simulink model "test_mashinka_mapp_4"  (R2020b)
settings: Solver=ode45  StartTime=0.0  StopTime=20000  RelTol=1e-3  EnableMultiTasking=on
undefined symbols (not defined in the file): CMD_ci_Re_9, CMD_fb, CMD_Firprg_0, CMD_Firprg_1, CMD_gain, CMD_ind_mult, CMD_ind_mult_1, CMD_ind_mult_2, CMD_ind_mult_3, CMD_ind_mult_4, CMD_ind_vol, CMD_ind_vol_1, CMD_ind_vol_2, CMD_ind_vol_3, CMD_ind_vol_4, CMD_nl, CMD_param_0, CMD_pedal, CMD_reset, CMD_shape_0, CMD_step_down, CMD_step_up, ind_mult_0, ind_mult_1, ind_mult_2, ind_mult_3, ind_mult_4, ind_mult_multiplier, num_harm_0, num_pts0, num_str0, num_str1, Res, rom_length
libraries: xbsIndex_r4 x2299
(part 2 of 11)

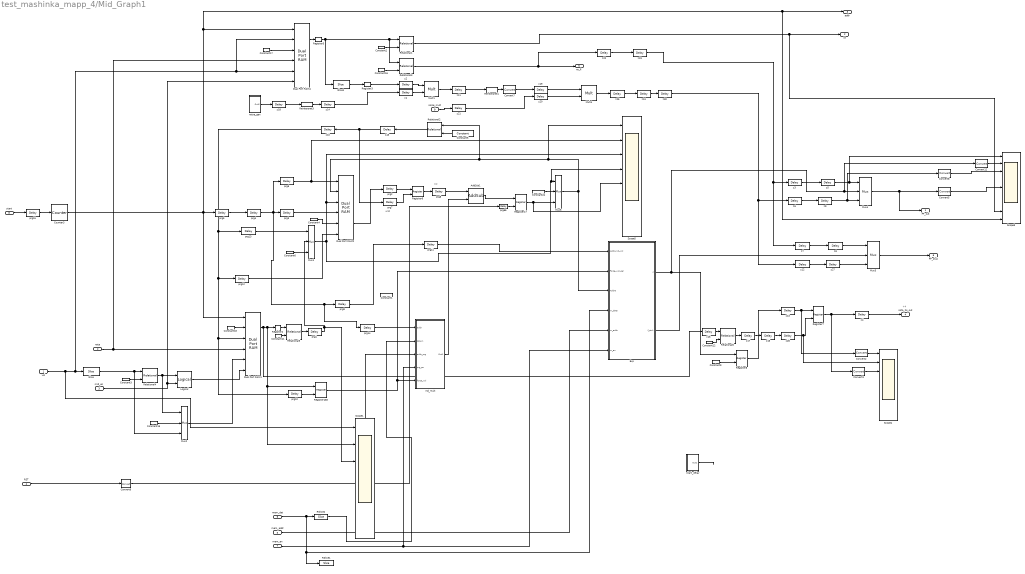
== system test_mashinka_mapp_4/Mid_Graph1 ==
  note: w90
  note: w2
  note: +4
  vol : Inport
  nota : Inport  Port=2
  mid_en : Inport  Port=3
  RST : Inport  Port=4
  mem_addr : Inport  Port=5
  mem_dat : Inport  Port=6
  mem_en : Inport  Port=7
  start : Inport  Port=8
  noise_mult : Inport  Port=9
  AddSub1 : xbsIndex_r4/AddSub  mode=Addition  use_carryin=off  use_carryout=off  en=off  latency=2  precision=User Defined  arith_type=Unsigned  n_bits=30  bin_pt=0  quantization=Truncate  overflow=Saturate  use_behavioral_HDL=off  hw_selection=Fabric  pipelined=off  dbl_ovrd=off  block_type=addsub
  Constant1 : xbsIndex_r4/Constant  const=4000  gui_display_data_type=Fixed-point  arith_type=Unsigned  n_bits=16  bin_pt=0  preci_type=Single  exp_width=8  frac_width=24  explicit_period=on  period=1  equ=P=C  opselect=C  inp2=PCIN>>17  opr=+  inp1=P  carry=CIN  dbl_ovrd=off  block_type=constant
      settings: block_version=VER_STRING_GOES_HERE
  Constant11 : xbsIndex_r4/Constant  const=1  gui_display_data_type=Fixed-point  arith_type=Unsigned  n_bits=7  bin_pt=0  preci_type=Single  exp_width=8  frac_width=24  explicit_period=on  period=1  equ=P=C  opselect=C  inp2=PCIN>>17  opr=+  inp1=P  carry=CIN  dbl_ovrd=off  block_type=constant
      settings: block_version=VER_STRING_GOES_HERE
  Constant{2,12,15,18} (4 alike) : xbsIndex_r4/Constant  const=0  gui_display_data_type=Fixed-point  arith_type=Unsigned  n_bits=7  bin_pt=0  preci_type=Single  exp_width=8  frac_width=24  explicit_period=on  period=1  equ=P=C  opselect=C  inp2=PCIN>>17  opr=+  inp1=P  carry=CIN  dbl_ovrd=off  block_type=constant
      settings: block_version=VER_STRING_GOES_HERE
  Constant16 : xbsIndex_r4/Constant  const=127  gui_display_data_type=Fixed-point  arith_type=Unsigned  n_bits=8  bin_pt=0  preci_type=Single  exp_width=8  frac_width=24  explicit_period=on  period=1  equ=P=C  opselect=C  inp2=PCIN>>17  opr=+  inp1=P  carry=CIN  dbl_ovrd=off  block_type=constant
      settings: block_version=VER_STRING_GOES_HERE
  Constant17 : xbsIndex_r4/Constant  const=0  gui_display_data_type=Fixed-point  arith_type=Boolean  n_bits=1  bin_pt=0  preci_type=Single  exp_width=8  frac_width=24  explicit_period=on  period=1  equ=P=C  opselect=C  inp2=PCIN>>17  opr=+  inp1=P  carry=CIN  dbl_ovrd=off  block_type=constant
      settings: block_version=VER_STRING_GOES_HERE
  Constant24 : xbsIndex_r4/Constant  const=0  gui_display_data_type=Fixed-point  arith_type=Unsigned  n_bits=30  bin_pt=0  preci_type=Single  exp_width=8  frac_width=24  explicit_period=on  period=1  equ=P=C  opselect=C  inp2=PCIN>>17  opr=+  inp1=P  carry=CIN  dbl_ovrd=off  block_type=constant
      settings: block_version=VER_STRING_GOES_HERE
  Constant3 : xbsIndex_r4/Constant  const=1  gui_display_data_type=Fixed-point  arith_type=Unsigned  n_bits=7  bin_pt=0  preci_type=Single  exp_width=8  frac_width=24  explicit_period=on  period=1  equ=P=C  opselect=C  inp2=PCIN>>17  opr=+  inp1=P  carry=CIN  dbl_ovrd=off  block_type=constant
      settings: block_version=VER_STRING_GOES_HERE
  Constant4 : xbsIndex_r4/Constant  const=0  gui_display_data_type=Fixed-point  arith_type=Unsigned  n_bits=30  bin_pt=0  preci_type=Single  exp_width=8  frac_width=24  explicit_period=on  period=1  equ=P=C  opselect=C  inp2=PCIN>>17  opr=+  inp1=P  carry=CIN  dbl_ovrd=off  block_type=constant
      settings: block_version=VER_STRING_GOES_HERE
  Constant5 : xbsIndex_r4/Constant  const=1000000000  gui_display_data_type=Fixed-point  arith_type=Unsigned  n_bits=30  bin_pt=0  preci_type=Single  exp_width=8  frac_width=24  explicit_period=off  period=1  equ=P=C  opselect=C  inp2=PCIN>>17  opr=+  inp1=P  carry=CIN  dbl_ovrd=off  block_type=constant
      settings: block_version=VER_STRING_GOES_HERE
  Constant6 : xbsIndex_r4/Constant  const=0  gui_display_data_type=Boolean  arith_type=Boolean  n_bits=24  bin_pt=0  preci_type=Single  exp_width=8  frac_width=24  explicit_period=on  period=1  equ=P=C  opselect=C  inp2=PCIN>>17  opr=+  inp1=P  carry=CIN  dbl_ovrd=off  block_type=constant
      settings: block_version=VER_STRING_GOES_HERE
  Constant9 : xbsIndex_r4/Constant  const=1  gui_display_data_type=Boolean  arith_type=Boolean  n_bits=24  bin_pt=0  preci_type=Single  exp_width=8  frac_width=24  explicit_period=on  period=1  equ=P=C  opselect=C  inp2=PCIN>>17  opr=+  inp1=P  carry=CIN  dbl_ovrd=off  block_type=constant
      settings: block_version=VER_STRING_GOES_HERE
  Convert{2..3,5,8,12} (5 alike) : xbsIndex_r4/Convert  gui_display_data_type=Floating-point  arith_type=Floating-point  n_bits=48  bin_pt=0  float_type=Single  exp_bits=8  fraction_bits=24  quantization="Round  (unbiased: +/- Inf)"  overflow=Saturate  en=off  latency=0  pipeline=off  dbl_ovrd=off  block_type=convert
  Convert6 : xbsIndex_r4/Convert  gui_display_data_type=Fixed-point  arith_type=Boolean  n_bits=48  bin_pt=48  float_type=Single  exp_bits=8  fraction_bits=24  quantization=Truncate  overflow=Saturate  en=off  latency=0  pipeline=off  dbl_ovrd=off  block_type=convert
      settings: xl_area=[0 0 0 0 0 0 0]  block_version=8.2-EVAL
  Convert7 : xbsIndex_r4/Convert  gui_display_data_type=Floating-point  arith_type=Floating-point  n_bits=48  bin_pt=0  float_type=Single  exp_bits=8  fraction_bits=24  quantization="Round  (unbiased: +/- Inf)"  overflow=Saturate  en=off  latency=6  pipeline=off  dbl_ovrd=off  block_type=convert
  Counter3 : xbsIndex_r4/Counter  cnt_type=Count Limited  cnt_to=95  operation=Up  start_count=0  cnt_by_val=1  arith_type=Unsigned  n_bits=7  bin_pt=0  load_pin=off  rst=off  en=on  explicit_period=on  period=1  use_behavioral_HDL=off  implementation=Fabric  use_rpm=off  dbl_ovrd=off  block_type=counter
      settings: block_version=8.2.02
  Dual Port RAM1 : xbsIndex_r4/Dual Port RAM  depth=96  initVector=zeros  distributed_mem=Block RAM  init_a=0  init_b=0  rst_a=off  rst_b=off  en_a=off  en_b=off  latency=1  write_mode_A=Read Before Write  write_mode_B=Read After Write  optimize=Area  dbl_ovrd=off  simulation_type=fast_sim  block_type=dpram
      settings: block_version=10.1.1
  Dual Port RAM2 : xbsIndex_r4/Dual Port RAM  depth=96  initVector=zeros  distributed_mem=Block RAM  init_a=0  init_b=0  rst_a=off  rst_b=off  en_a=off  en_b=off  latency=1  write_mode_A=Read Before Write  write_mode_B=Read After Write  optimize=Area  dbl_ovrd=off  simulation_type=fast_sim  block_type=dpram
      settings: block_version=10.1.1
  Dual Port RAM4 : xbsIndex_r4/Dual Port RAM  depth=96  initVector=zeros  distributed_mem=Block RAM  init_a=0  init_b=0  rst_a=off  rst_b=off  en_a=off  en_b=off  latency=1  write_mode_A=Read Before Write  write_mode_B=Read After Write  optimize=Area  dbl_ovrd=off  simulation_type=fast_sim  block_type=dpram
      settings: block_version=10.1.1
  Exp : Subsystem
  Logical : xbsIndex_r4/Logical  logical_function=AND  inputs=2  en=off  latency=0  precision=Full  arith_type=Unsigned  n_bits=16  bin_pt=0  align_bp=on  dbl_ovrd=off  block_type=logical
  Mult1 : xbsIndex_r4/Mult  precision=Full  arith_type="Signed  (2's comp)"  n_bits=16  bin_pt=14  quantization=Truncate  overflow=Wrap  en=off  latency=6  use_behavioral_HDL=off  opt=Speed  use_embedded=on  optimum_pipeline=off  pipeline=on  dbl_ovrd=off  use_rpm=on  placement_style=Triangular  block_type=mult
  Mult4 : xbsIndex_r4/Mult  precision=Full  arith_type="Signed  (2's comp)"  n_bits=16  bin_pt=14  quantization=Truncate  overflow=Wrap  en=off  latency=6  use_behavioral_HDL=off  opt=Speed  use_embedded=on  optimum_pipeline=off  pipeline=on  dbl_ovrd=off  use_rpm=on  placement_style=Triangular  block_type=mult
  Mux{1..5} (5 alike) : xbsIndex_r4/Mux  inputs=2  en=off  latency=0  precision=Full  arith_type=Unsigned  n_bits=16  bin_pt=14  quantization=Truncate  overflow=Wrap  dbl_ovrd=off  block_type=mux
  RSlice1 : xbsIndex_r4/Slice  nbits=30  boolean_output=off  mode=Lower Bit Location + Width  bit1=0  base1=MSB of Input  bit0=0  base0=LSB of Input  dbl_ovrd=off  block_type=slice
      settings: block_version=VER_STRING_GOES_HERE
  RSlice2 : xbsIndex_r4/Slice  nbits=24  boolean_output=off  mode=Lower Bit Location + Width  bit1=0  base1=MSB of Input  bit0=0  base0=LSB of Input  dbl_ovrd=off  block_type=slice
      settings: block_version=VER_STRING_GOES_HERE
  Register17 : xbsIndex_r4/Register  init=0  rst=on  en=off  dbl_ovrd=off  block_type=register
  Register183 : xbsIndex_r4/Register  init=0  rst=on  en=off  dbl_ovrd=off  block_type=register
  Register2 : xbsIndex_r4/Register  init=0  rst=off  en=off  dbl_ovrd=off  block_type=register
  Register3 : xbsIndex_r4/Register  init=0  rst=off  en=off  dbl_ovrd=off  block_type=register
  Register5 : xbsIndex_r4/Register  init=0  rst=off  en=off  dbl_ovrd=off  block_type=register
  Register6 : xbsIndex_r4/Register  init=0  rst=on  en=off  dbl_ovrd=off  block_type=register
  Register7 : xbsIndex_r4/Register  init=1  rst=off  en=on  dbl_ovrd=off  block_type=register
  Register8 : xbsIndex_r4/Register  init=0  rst=off  en=on  dbl_ovrd=off  block_type=register
  Reinterpret1 : xbsIndex_r4/Reinterpret  force_arith_type=on  arith_type="Signed  (2's comp)"  force_bin_pt=on  bin_pt=30  block_type=reinterpret
  Reinterpret3 : xbsIndex_r4/Reinterpret  force_arith_type=on  arith_type="Signed  (2's comp)"  force_bin_pt=on  bin_pt=0  block_type=reinterpret
  Relational{1,3..6} (5 alike) : xbsIndex_r4/Relational  mode=a>b  op_type=Bool  en=off  latency=0  dbl_ovrd=off  block_type=relational
  Relational2 : xbsIndex_r4/Relational  mode=a>=b  op_type=Bool  en=off  latency=0  dbl_ovrd=off  block_type=relational
  Scope1 : Scope  NumInputPorts=7
  Scope3 : Scope  NumInputPorts=9
  Scope4 : Scope  NumInputPorts=8
  Scope5 : Scope  NumInputPorts=8
  Slice : xbsIndex_r4/Slice  nbits=7  boolean_output=off  mode=Lower Bit Location + Width  bit1=0  base1=MSB of Input  bit0=0  base0=LSB of Input  dbl_ovrd=off  block_type=slice
  Slice1 : xbsIndex_r4/Slice  nbits=7  boolean_output=off  mode=Lower Bit Location + Width  bit1=0  base1=MSB of Input  bit0=0  base0=LSB of Input  dbl_ovrd=off  block_type=slice
  ind_mult : Subsystem
  noise_gen : Subsystem
  prg1 : xbsIndex_r4/Delay  rst=off  infoeditControl=Selection of Reset will increase slice count due to use of real FFs and instead of SRLs  en=off  latency=12  reg_retiming=on  dbl_ovrd=off  block_type=delay
      settings: block_version=8.2-EVAL
  prg10 : xbsIndex_r4/Delay  rst=off  infoeditControl=Selection of Reset will increase slice count due to use of real FFs and instead of SRLs  en=off  latency=8  reg_retiming=on  dbl_ovrd=off  block_type=delay
      settings: block_version=8.2-EVAL
  prg11 : xbsIndex_r4/Delay  rst=off  infoeditControl=Selection of Reset will increase slice count due to use of real FFs and instead of SRLs  en=off  latency=2  reg_retiming=on  dbl_ovrd=off  block_type=delay
      settings: block_version=8.2-EVAL
  prg12 : xbsIndex_r4/Delay  rst=off  infoeditControl=Selection of Reset will increase slice count due to use of real FFs and instead of SRLs  en=off  latency=6  reg_retiming=on  dbl_ovrd=off  block_type=delay
      settings: block_version=8.2-EVAL
  prg13 : xbsIndex_r4/Delay  rst=off  infoeditControl=Selection of Reset will increase slice count due to use of real FFs and instead of SRLs  en=off  latency=14  reg_retiming=on  dbl_ovrd=off  block_type=delay
      settings: block_version=8.2-EVAL
  prg14 : xbsIndex_r4/Delay  rst=off  infoeditControl=Selection of Reset will increase slice count due to use of real FFs and instead of SRLs  en=off  latency=6  reg_retiming=on  dbl_ovrd=off  block_type=delay
      settings: block_version=8.2-EVAL
  prg{2,4,15,66} (4 alike) : xbsIndex_r4/Delay  rst=off  infoeditControl=Selection of Reset will increase slice count due to use of real FFs and instead of SRLs  en=off  latency=1  reg_retiming=on  dbl_ovrd=off  block_type=delay
      settings: block_version=8.2-EVAL
  prg3 : xbsIndex_r4/Delay  rst=off  infoeditControl=Selection of Reset will increase slice count due to use of real FFs and instead of SRLs  en=off  latency=8 + 7  reg_retiming=on  dbl_ovrd=off  block_type=delay
      settings: block_version=8.2-EVAL
  prg5 : xbsIndex_r4/Delay  rst=off  infoeditControl=Selection of Reset will increase slice count due to use of real FFs and instead of SRLs  en=off  latency=86  reg_retiming=on  dbl_ovrd=off  block_type=delay
      settings: block_version=8.2-EVAL
  prg6 : xbsIndex_r4/Delay  rst=off  infoeditControl=Selection of Reset will increase slice count due to use of real FFs and instead of SRLs  en=off  latency=16 + 7  reg_retiming=on  dbl_ovrd=off  block_type=delay
      settings: block_version=8.2-EVAL
  prg7 : xbsIndex_r4/Delay  rst=off  infoeditControl=Selection of Reset will increase slice count due to use of real FFs and instead of SRLs  en=off  latency=93 - 6  reg_retiming=on  dbl_ovrd=off  block_type=delay
      settings: block_version=8.2-EVAL
  prg8 : xbsIndex_r4/Delay  rst=off  infoeditControl=Selection of Reset will increase slice count due to use of real FFs and instead of SRLs  en=off  latency=2  reg_retiming=on  dbl_ovrd=off  block_type=delay
      settings: block_version=8.2-EVAL
  prg9 : xbsIndex_r4/Delay  rst=off  infoeditControl=Selection of Reset will increase slice count due to use of real FFs and instead of SRLs  en=off  latency=8  reg_retiming=on  dbl_ovrd=off  block_type=delay
      settings: block_version=8.2-EVAL
  start_delay : Subsystem
  z{1..2,4..5,8..9,11,13..14,16..21,23,25..27,30} (20 alike) : xbsIndex_r4/Delay  rst=off  infoeditControl=Selection of Reset will increase slice count due to use of real FFs and instead of SRLs  en=off  latency=1  reg_retiming=on  dbl_ovrd=off  block_type=delay
      settings: block_version=8.2-EVAL
  z10 : xbsIndex_r4/Delay  rst=off  infoeditControl=Selection of Reset will increase slice count due to use of real FFs and instead of SRLs  en=off  latency=86 -7  reg_retiming=on  dbl_ovrd=off  block_type=delay
      settings: block_version=8.2-EVAL
  z{3,6..7,12} (4 alike) : xbsIndex_r4/Delay  rst=off  infoeditControl=Selection of Reset will increase slice count due to use of real FFs and instead of SRLs  en=off  latency=35 + 7  reg_retiming=on  dbl_ovrd=off  block_type=delay
      settings: block_version=8.2-EVAL
  z15 : xbsIndex_r4/Delay  rst=off  infoeditControl=Selection of Reset will increase slice count due to use of real FFs and instead of SRLs  en=off  latency=98  reg_retiming=on  dbl_ovrd=off  block_type=delay
      settings: block_version=8.2-EVAL
  z22 : xbsIndex_r4/Delay  rst=off  infoeditControl=Selection of Reset will increase slice count due to use of real FFs and instead of SRLs  en=off  latency=54  reg_retiming=on  dbl_ovrd=off  block_type=delay
      settings: block_version=8.2-EVAL
  z24 : xbsIndex_r4/Delay  rst=off  infoeditControl=Selection of Reset will increase slice count due to use of real FFs and instead of SRLs  en=off  latency=31  reg_retiming=on  dbl_ovrd=off  block_type=delay
      settings: block_version=8.2-EVAL
  z43 : xbsIndex_r4/Delay  rst=off  infoeditControl=Selection of Reset will increase slice count due to use of real FFs and instead of SRLs  en=off  latency=3  reg_retiming=on  dbl_ovrd=off  block_type=delay
      settings: block_version=8.2-EVAL
  FF_out : Outport  VectorParamsAs1DForOutWhenUnconnected=off
  nn : Outport  Port=2  VectorParamsAs1DForOutWhenUnconnected=off
  addr : Outport  Port=3  VectorParamsAs1DForOutWhenUnconnected=off
  nota_24_out : Outport  Port=4  VectorParamsAs1DForOutWhenUnconnected=off
  nn_fl : Outport  Port=5  VectorParamsAs1DForOutWhenUnconnected=off
  FF_stuk : Outport  Port=6  VectorParamsAs1DForOutWhenUnconnected=off
  wires:
  z5/1 -> Mux4/1, Scope3/1
  Convert3/1 -> Scope4/3
  Convert2/1 -> Scope4/1
  Constant12/1 -> Relational6/2
  Constant9/1 -> Register8/2
  z13/1 -> Register7/1, Convert2/1
  Relational6/1 -> z17/1
  z15/1 -> z26/1
  z16/1 -> Relational6/1
  z17/1 -> z15/1
  z26/1 -> Register7/2, Scope4/2
  Register8/1 -> z13/1
  Convert12/1 -> Scope3/2
  Convert8/1 -> Scope3/3
  Convert5/1 -> Scope3/5
  Mux4/1 -> Convert5/1, FF_out/1
  z9/1 -> Mux4/3, Convert8/1
  z3/1 -> z5/1
  Counter3/1 -> prg5/1, Dual Port RAM1/1, addr/1, Scope3/9, Dual Port RAM4/1
  mem_dat/1 -> RSlice2/1, RSlice1/1, Exp/4(m_data)
  Exp/1(f) -> Mux4/2, Convert12/1, Register8/1
  z30/1 -> z12/1, z6/1
  z25/1 -> z24/1
  z24/1 -> z30/1
  z23/1 -> z7/1, z3/1
  z22/1 -> z23/1
  Mult4/1 -> z25/1
  z21/1 -> z20/1
  noise_mult/1 -> z21/1
  Mult1/1 -> z11/1
  z19/1 -> Mult4/1
  z11/1 -> Reinterpret1/1
  Convert7/1 -> z19/1
  Reinterpret1/1 -> Convert7/1
  z20/1 -> Mult4/2
  Register3/1 -> z2/1
  z2/1 -> Mult1/1
  z1/1 -> Mult1/2
  Slice1/1 -> Register3/1
  Reinterpret3/1 -> z14/1
  z14/1 -> z1/1
  Relational3/1 -> nn_fl/1, z22/1
  Constant16/1 -> Relational3/2
  vol/1 -> Slice/1, Dual Port RAM4/5, Dual Port RAM4/2, Scope1/1
  Slice/1 -> Mux2/3, Relational4/1
  prg3/1 -> Dual Port RAM2/4
  prg1/1 -> Mux1/2, Scope1/3
  Constant6/1 -> Mux1/3
  prg13/1 -> Mux1/1
  Constant4/1 -> Dual Port RAM2/5
  prg12/1 -> Dual Port RAM2/6
  z4/1 -> nota_24_out/1
  prg5/1 -> prg4/1
  Logical/1 -> Dual Port RAM1/6
  prg11/1 -> Exp/1(Addr_ind_vol)
  z10/1 -> prg12/1, Dual Port RAM1/3, prg10/1, prg13/1
  Dual Port RAM1/1 -> Register2/1, Register183/1, Scope1/2, z16/1
  Relational5/1 -> prg1/1
  prg4/1 -> prg14/1, prg9/1, prg3/1, prg6/1
  prg6/1 -> Dual Port RAM2/1, Scope5/2
  Register5/1 -> Relational1/1, Relational3/1, Slice1/1
  prg2/1 -> Register6/1
  Dual Port RAM2/2 -> prg2/1
  Constant17/1 -> Dual Port RAM4/3
  Dual Port RAM4/1 -> Register5/1
  Register6/1 -> prg8/1
  Constant18/1 -> Dual Port RAM1/2
  prg7/1 -> Register6/2
  prg10/1 -> Register183/2
  Constant2/1 -> Relational1/2
  Relational1/1 -> nn/1, Scope3/8
  Constant5/1 -> Relational2/2
  z43/1 -> z10/1, prg7/1
  Relational2/1 -> z43/1
  Constant3/1 -> Relational4/2
  Relational4/1 -> Mux2/1, Logical/1
  Constant11/1 -> Relational5/2
  Register2/1 -> Relational5/1
  AddSub1/1 -> Register17/1
  RST/1 -> Convert6/1
  Convert6/1 -> prg66/1
  prg66/1 -> Register17/2
  Mux5/1 -> Scope5/1, Relational2/1, Dual Port RAM2/2, Exp/3(Addr0)
  Register17/1 -> Mux5/3, Scope5/5
  Constant24/1 -> Mux5/2
  Mux1/1 -> Dual Port RAM2/3, Scope5/3, Mux5/1, Scope5/4
  mem_en/1 -> Exp/6(m_en), ind_mult/4(prg_en)
  mem_addr/1 -> Exp/5(m_addr), ind_mult/3(addr_prg)
  RSlice2/1 -> ind_mult/2(dat_in)
  Register183/1 -> Exp/2(Force_vol_sel), ind_mult/5(force_vol)
  ind_mult/1(Out1) -> AddSub1/2
  prg9/1 -> prg11/1
  prg8/1 -> AddSub1/1
  start_delay/1(Out1) -> ?
  prg14/1 -> ind_mult/1(addr)
  start/1 -> prg15/1
  prg15/1 -> Counter3/1
  mid_en/1 -> Dual Port RAM4/6, Logical/2
  nota/1 -> Dual Port RAM4/4, Dual Port RAM1/4
  z18/1 -> Reinterpret3/1
  Constant15/1 -> Mux2/2
  Mux2/1 -> Dual Port RAM1/5
  noise_gen/1(Out2) -> z18/1
  Register7/1 -> z4/1, Convert3/1
  z6/1 -> z9/1
  z12/1 -> z27/1
  Exp/2(f_stuk) -> Mux3/2
  z7/1 -> z8/1
  z27/1 -> Mux3/3
  Mux3/1 -> FF_stuk/1
  z8/1 -> Mux3/1

== system test_mashinka_mapp_4/Reciever16 ==
  s_dat : Inport
  clk : Inport  Port=2
  frm : Inport  Port=3
  Convert : xbsIndex_r4/Convert  gui_display_data_type=Fixed-point  arith_type=Boolean  n_bits=16  bin_pt=14  float_type=Single  exp_bits=8  fraction_bits=24  quantization=Truncate  overflow=Wrap  en=off  latency=0  pipeline=off  dbl_ovrd=off  block_type=convert
      settings: xl_area=[0 0 0 0 0 0 0]  block_version=8.2-EVAL
  Convert1 : xbsIndex_r4/Convert  gui_display_data_type=Boolean  arith_type=Boolean  n_bits=16  bin_pt=14  float_type=Single  exp_bits=8  fraction_bits=24  quantization=Truncate  overflow=Wrap  en=off  latency=0  pipeline=off  dbl_ovrd=off  block_type=convert
      settings: xl_area=[0 0 0 0 0 0 0]  block_version=8.2-EVAL
  Delay : xbsIndex_r4/Delay  rst=off  infoeditControl=Selection of Reset will increase slice count due to use of real FFs and instead of SRLs  en=off  latency=1  reg_retiming=on  dbl_ovrd=off  block_type=delay
      settings: infoedit=Hardware notes: A delay line is a chain, each link of which is an SRL16 followed by a flip-flop. If register retiming is enabled, the delay line is a chain of flip-flops.  xl_area=[1 1 0 0 0 0 0]  block_version=8.2-EVAL
  Delay1 : xbsIndex_r4/Delay  rst=off  infoeditControl=Selection of Reset will increase slice count due to use of real FFs and instead of SRLs  en=off  latency=5  reg_retiming=on  dbl_ovrd=off  block_type=delay
      settings: infoedit=Hardware notes: A delay line is a chain, each link of which is an SRL16 followed by a flip-flop. If register retiming is enabled, the delay line is a chain of flip-flops.  xl_area=[1 1 0 1 0 0 0]  block_version=8.2-EVAL
  Delay2 : xbsIndex_r4/Delay  rst=off  infoeditControl=Selection of Reset will increase slice count due to use of real FFs and instead of SRLs  en=off  latency=1  reg_retiming=on  dbl_ovrd=off  block_type=delay
      settings: infoedit=Hardware notes: A delay line is a chain, each link of which is an SRL16 followed by a flip-flop. If register retiming is enabled, the delay line is a chain of flip-flops.  xl_area=[1 1 0 0 0 0 0]  block_version=8.2-EVAL
  Delay3 : xbsIndex_r4/Delay  rst=off  infoeditControl=Selection of Reset will increase slice count due to use of real FFs and instead of SRLs  en=off  latency=7  reg_retiming=on  dbl_ovrd=off  block_type=delay
      settings: infoedit=Hardware notes: A delay line is a chain, each link of which is an SRL16 followed by a flip-flop. If register retiming is enabled, the delay line is a chain of flip-flops.  xl_area=[1 1 0 1 0 0 0]  block_version=8.2-EVAL
  Delay4 : xbsIndex_r4/Delay  rst=off  infoeditControl=Selection of Reset will increase slice count due to use of real FFs and instead of SRLs  en=off  latency=3  reg_retiming=on  dbl_ovrd=off  block_type=delay
      settings: infoedit=Hardware notes: A delay line is a chain, each link of which is an SRL16 followed by a flip-flop. If register retiming is enabled, the delay line is a chain of flip-flops.  xl_area=[1 1 0 0 0 0 0]  block_version=8.2-EVAL
  Delay5 : xbsIndex_r4/Delay  rst=off  infoeditControl=Selection of Reset will increase slice count due to use of real FFs and instead of SRLs  en=off  latency=1  reg_retiming=on  dbl_ovrd=off  block_type=delay
      settings: infoedit=Hardware notes: A delay line is a chain, each link of which is an SRL16 followed by a flip-flop. If register retiming is enabled, the delay line is a chain of flip-flops.  xl_area=[1 1 0 0 0 0 0]  block_version=8.2-EVAL
  Inverter : xbsIndex_r4/Inverter  en=off  latency=0  dbl_ovrd=off  block_type=inv
      settings: xl_area=[0 0 0 0 0 0 0]  block_version=8.2-EVAL
  Logical : xbsIndex_r4/Logical  logical_function=XOR  inputs=2  en=off  latency=0  precision=Full  arith_type=Unsigned  n_bits=16  bin_pt=0  align_bp=on  dbl_ovrd=off  block_type=logical
      settings: xl_area=[1 0 0 1 0 0 0]  block_version=8.2-EVAL
  Logical1 : xbsIndex_r4/Logical  logical_function=AND  inputs=2  en=off  latency=0  precision=Full  arith_type=Unsigned  n_bits=16  bin_pt=0  align_bp=on  dbl_ovrd=off  block_type=logical
      settings: xl_area=[1 0 0 1 0 0 0]  block_version=8.2-EVAL
  Scope : Scope  NumInputPorts=4
  Subsystem1 : Subsystem
  Z1 : Subsystem
  Out1 : Outport  VectorParamsAs1DForOutWhenUnconnected=off
  reset_z1 : Outport  Port=2  VectorParamsAs1DForOutWhenUnconnected=off
  wires:
  frm/1 -> Delay3/1
  clk/1 -> Delay2/1
  s_dat/1 -> Delay1/1
  Delay/1 -> Logical/1
  Logical/1 -> Logical1/1
  Logical1/1 -> Convert/1
  Convert/1 -> Scope/3, Subsystem1/2(en), Delay4/1, Delay5/1
  Delay1/1 -> Scope/1, Subsystem1/1(data)
  Delay2/1 -> Z1/1(In1)
  Convert1/1 -> Scope/2, Subsystem1/3(clock)
  Z1/1(Out1) -> Convert1/1
  Inverter/1 -> Logical1/2
  Delay3/1 -> Logical/2, Inverter/1, Delay/1
  Delay4/1 -> Subsystem1/4(reset)
  Subsystem1/1(Out1) -> Scope/4, Out1/1
  Delay5/1 -> reset_z1/1

== system test_mashinka_mapp_4/Reciever50 ==
  s_dat : Inport
  clk : Inport  Port=2
  frm : Inport  Port=3
  Convert : xbsIndex_r4/Convert  gui_display_data_type=Fixed-point  arith_type=Boolean  n_bits=16  bin_pt=14  float_type=Single  exp_bits=8  fraction_bits=24  quantization=Truncate  overflow=Wrap  en=off  latency=0  pipeline=off  dbl_ovrd=off  block_type=convert
      settings: xl_area=[0 0 0 0 0 0 0]  block_version=8.2-EVAL
  Convert1 : xbsIndex_r4/Convert  gui_display_data_type=Boolean  arith_type=Boolean  n_bits=16  bin_pt=14  float_type=Single  exp_bits=8  fraction_bits=24  quantization=Truncate  overflow=Wrap  en=off  latency=0  pipeline=off  dbl_ovrd=off  block_type=convert
      settings: xl_area=[0 0 0 0 0 0 0]  block_version=8.2-EVAL
  Delay : xbsIndex_r4/Delay  rst=off  infoeditControl=Selection of Reset will increase slice count due to use of real FFs and instead of SRLs  en=off  latency=1  reg_retiming=on  dbl_ovrd=off  block_type=delay
      settings: infoedit=Hardware notes: A delay line is a chain, each link of which is an SRL16 followed by a flip-flop. If register retiming is enabled, the delay line is a chain of flip-flops.  xl_area=[1 1 0 0 0 0 0]  block_version=8.2-EVAL
  Delay1 : xbsIndex_r4/Delay  rst=off  infoeditControl=Selection of Reset will increase slice count due to use of real FFs and instead of SRLs  en=off  latency=5  reg_retiming=on  dbl_ovrd=off  block_type=delay
      settings: infoedit=Hardware notes: A delay line is a chain, each link of which is an SRL16 followed by a flip-flop. If register retiming is enabled, the delay line is a chain of flip-flops.  xl_area=[1 1 0 1 0 0 0]  block_version=8.2-EVAL
  Delay2 : xbsIndex_r4/Delay  rst=off  infoeditControl=Selection of Reset will increase slice count due to use of real FFs and instead of SRLs  en=off  latency=1  reg_retiming=on  dbl_ovrd=off  block_type=delay
      settings: infoedit=Hardware notes: A delay line is a chain, each link of which is an SRL16 followed by a flip-flop. If register retiming is enabled, the delay line is a chain of flip-flops.  xl_area=[1 1 0 0 0 0 0]  block_version=8.2-EVAL
  Delay3 : xbsIndex_r4/Delay  rst=off  infoeditControl=Selection of Reset will increase slice count due to use of real FFs and instead of SRLs  en=off  latency=7  reg_retiming=on  dbl_ovrd=off  block_type=delay
      settings: infoedit=Hardware notes: A delay line is a chain, each link of which is an SRL16 followed by a flip-flop. If register retiming is enabled, the delay line is a chain of flip-flops.  xl_area=[1 1 0 1 0 0 0]  block_version=8.2-EVAL
  Delay4 : xbsIndex_r4/Delay  rst=off  infoeditControl=Selection of Reset will increase slice count due to use of real FFs and instead of SRLs  en=off  latency=3  reg_retiming=on  dbl_ovrd=off  block_type=delay
      settings: infoedit=Hardware notes: A delay line is a chain, each link of which is an SRL16 followed by a flip-flop. If register retiming is enabled, the delay line is a chain of flip-flops.  xl_area=[1 1 0 0 0 0 0]  block_version=8.2-EVAL
  Delay5 : xbsIndex_r4/Delay  rst=off  infoeditControl=Selection of Reset will increase slice count due to use of real FFs and instead of SRLs  en=off  latency=1  reg_retiming=on  dbl_ovrd=off  block_type=delay
      settings: infoedit=Hardware notes: A delay line is a chain, each link of which is an SRL16 followed by a flip-flop. If register retiming is enabled, the delay line is a chain of flip-flops.  xl_area=[1 1 0 0 0 0 0]  block_version=8.2-EVAL
  Inverter : xbsIndex_r4/Inverter  en=off  latency=0  dbl_ovrd=off  block_type=inv
      settings: xl_area=[0 0 0 0 0 0 0]  block_version=8.2-EVAL
  Logical : xbsIndex_r4/Logical  logical_function=XOR  inputs=2  en=off  latency=0  precision=Full  arith_type=Unsigned  n_bits=16  bin_pt=0  align_bp=on  dbl_ovrd=off  block_type=logical
      settings: xl_area=[1 0 0 1 0 0 0]  block_version=8.2-EVAL
  Logical1 : xbsIndex_r4/Logical  logical_function=AND  inputs=2  en=off  latency=0  precision=Full  arith_type=Unsigned  n_bits=16  bin_pt=0  align_bp=on  dbl_ovrd=off  block_type=logical
      settings: xl_area=[1 0 0 1 0 0 0]  block_version=8.2-EVAL
  Scope : Scope  NumInputPorts=4
  Subsystem1 : Subsystem
  Z1 : Subsystem
  Out1 : Outport  VectorParamsAs1DForOutWhenUnconnected=off
  reset_z1 : Outport  Port=2  VectorParamsAs1DForOutWhenUnconnected=off
  wires:
  Delay5/1 -> reset_z1/1
  Subsystem1/1(Out1) -> Out1/1, Scope/4
  Delay4/1 -> Subsystem1/4(reset)
  Delay3/1 -> Delay/1, Inverter/1, Logical/2
  Inverter/1 -> Logical1/2
  Z1/1(Out1) -> Convert1/1
  Convert1/1 -> Subsystem1/3(clock), Scope/2
  Delay2/1 -> Z1/1(In1)
  Delay1/1 -> Subsystem1/1(data), Scope/1
  Convert/1 -> Delay5/1, Delay4/1, Subsystem1/2(en), Scope/3
  Logical1/1 -> Convert/1
  Logical/1 -> Logical1/1
  Delay/1 -> Logical/1
  s_dat/1 -> Delay1/1
  clk/1 -> Delay2/1
  frm/1 -> Delay3/1

== system test_mashinka_mapp_4/SIMULATION ==
  Accumulator : xbsIndex_r4/Accumulator  operation=Add  n_bits=3  overflow=Wrap  scale=1  rst=off  hasbypass=off  infoeditControl=reset for floating point data type must be asserted for a minimum of 2 cycles  en=on  latency=1  msb_inp=100  msb=100  lsb=-100  use_behavioral_HDL=on  implementation=Fabric  dbl_ovrd=off  block_type=accum
      settings: block_version=11.4
  Concat{1..6} (6 alike) : xbsIndex_r4/Concat  num_inputs=2  dbl_ovrd=off  block_type=concat
  Constant1 : xbsIndex_r4/Constant  const=60000  gui_display_data_type=Fixed-point  arith_type=Unsigned  n_bits=18  bin_pt=0  preci_type=Single  exp_width=8  frac_width=24  explicit_period=on  period=1  equ=P=C  opselect=C  inp2=PCIN>>17  opr=+  inp1=P  carry=CIN  dbl_ovrd=off  block_type=constant
      settings: block_version=8.2-EVAL
  Constant10 : xbsIndex_r4/Constant  const=1  gui_display_data_type=Boolean  arith_type=Boolean  n_bits=18  bin_pt=0  preci_type=Single  exp_width=8  frac_width=24  explicit_period=on  period=1  equ=P=C  opselect=C  inp2=PCIN>>17  opr=+  inp1=P  carry=CIN  dbl_ovrd=off  block_type=constant
      settings: block_version=8.2-EVAL
  Constant2 : xbsIndex_r4/Constant  const=700000  gui_display_data_type=Fixed-point  arith_type=Unsigned  n_bits=18  bin_pt=0  preci_type=Single  exp_width=8  frac_width=24  explicit_period=on  period=1  equ=P=C  opselect=C  inp2=PCIN>>17  opr=+  inp1=P  carry=CIN  dbl_ovrd=off  block_type=constant
      settings: block_version=8.2-EVAL
  Constant3 : xbsIndex_r4/Constant  const=1500  gui_display_data_type=Fixed-point  arith_type=Unsigned  n_bits=18  bin_pt=0  preci_type=Single  exp_width=8  frac_width=24  explicit_period=on  period=1  equ=P=C  opselect=C  inp2=PCIN>>17  opr=+  inp1=P  carry=CIN  dbl_ovrd=off  block_type=constant
      settings: block_version=8.2-EVAL
  Constant4 : xbsIndex_r4/Constant  const=1  gui_display_data_type=Fixed-point  arith_type=Unsigned  n_bits=1  bin_pt=0  preci_type=Single  exp_width=8  frac_width=24  explicit_period=on  period=1  equ=P=C  opselect=C  inp2=PCIN>>17  opr=+  inp1=P  carry=CIN  dbl_ovrd=off  block_type=constant
      settings: block_version=8.2-EVAL
  Constant5 : xbsIndex_r4/Constant  const=1500  gui_display_data_type=Fixed-point  arith_type=Unsigned  n_bits=18  bin_pt=0  preci_type=Single  exp_width=8  frac_width=24  explicit_period=on  period=1  equ=P=C  opselect=C  inp2=PCIN>>17  opr=+  inp1=P  carry=CIN  dbl_ovrd=off  block_type=constant
      settings: block_version=8.2-EVAL
  Constant6 : xbsIndex_r4/Constant  const=2000  gui_display_data_type=Fixed-point  arith_type=Unsigned  n_bits=18  bin_pt=0  preci_type=Single  exp_width=8  frac_width=24  explicit_period=on  period=1  equ=P=C  opselect=C  inp2=PCIN>>17  opr=+  inp1=P  carry=CIN  dbl_ovrd=off  block_type=constant
      settings: block_version=8.2-EVAL
  Constant7 : xbsIndex_r4/Constant  const=2500  gui_display_data_type=Fixed-point  arith_type=Unsigned  n_bits=18  bin_pt=0  preci_type=Single  exp_width=8  frac_width=24  explicit_period=on  period=1  equ=P=C  opselect=C  inp2=PCIN>>17  opr=+  inp1=P  carry=CIN  dbl_ovrd=off  block_type=constant
      settings: block_version=8.2-EVAL
  Constant8 : xbsIndex_r4/Constant  const=3000  gui_display_data_type=Fixed-point  arith_type=Unsigned  n_bits=18  bin_pt=0  preci_type=Single  exp_width=8  frac_width=24  explicit_period=on  period=1  equ=P=C  opselect=C  inp2=PCIN>>17  opr=+  inp1=P  carry=CIN  dbl_ovrd=off  block_type=constant
      settings: block_version=8.2-EVAL
  Constant9 : xbsIndex_r4/Constant  const=1000  gui_display_data_type=Fixed-point  arith_type=Unsigned  n_bits=18  bin_pt=0  preci_type=Single  exp_width=8  frac_width=24  explicit_period=on  period=1  equ=P=C  opselect=C  inp2=PCIN>>17  opr=+  inp1=P  carry=CIN  dbl_ovrd=off  block_type=constant
      settings: block_version=8.2-EVAL
  Counter : xbsIndex_r4/Counter  cnt_type=Free Running  cnt_to=Inf  operation=Up  start_count=0  cnt_by_val=1  arith_type=Unsigned  n_bits=29  bin_pt=0  load_pin=off  rst=off  en=on  explicit_period=on  period=1  use_behavioral_HDL=off  implementation=Fabric  use_rpm=off  dbl_ovrd=off  block_type=counter
      settings: xl_area=[11 20 0 20 0 0 0]  block_version=8.2-EVAL
  Counter1 : xbsIndex_r4/Counter  cnt_type=Free Running  cnt_to=Inf  operation=Up  start_count=0  cnt_by_val=1  arith_type=Unsigned  n_bits=29  bin_pt=0  load_pin=off  rst=off  en=off  explicit_period=on  period=1  use_behavioral_HDL=off  implementation=Fabric  use_rpm=off  dbl_ovrd=off  block_type=counter
      settings: xl_area=[11 20 0 20 0 0 0]  block_version=8.2-EVAL
  Logical3 : xbsIndex_r4/Logical  logical_function=OR  inputs=6  en=off  latency=0  precision=Full  arith_type=Unsigned  n_bits=16  bin_pt=0  align_bp=on  dbl_ovrd=off  block_type=logical
      settings: xl_area=[1 0 0 1 0 0 0]  block_version=8.2-EVAL
  Logical7 : xbsIndex_r4/Logical  logical_function=OR  inputs=2  en=off  latency=0  precision=Full  arith_type=Unsigned  n_bits=16  bin_pt=0  align_bp=on  dbl_ovrd=off  block_type=logical
      settings: xl_area=[1 0 0 1 0 0 0]  block_version=8.2-EVAL
  Mux1 : xbsIndex_r4/Mux  inputs=6  en=off  latency=0  precision=Full  arith_type=Unsigned  n_bits=16  bin_pt=14  quantization=Truncate  overflow=Wrap  dbl_ovrd=off  block_type=mux
      settings: block_version=11.4
  Register1 : xbsIndex_r4/Register  init=0  rst=off  en=on  dbl_ovrd=off  block_type=register
      settings: block_version=8.2-EVAL
  Relational{1..3,9..13} (8 alike) : xbsIndex_r4/Relational  mode=a=b  op_type=Bool  en=off  latency=1  dbl_ovrd=off  block_type=relational
      settings: xl_area=[5 1 0 10 0 0 0]  block_version=8.2-EVAL
  Slice2 : xbsIndex_r4/Slice  nbits=8  boolean_output=off  mode=Lower Bit Location + Width  bit1=0  base1=MSB of Input  bit0=7  base0=LSB of Input  dbl_ovrd=off  block_type=slice
  Slice3 : xbsIndex_r4/Slice  nbits=7  boolean_output=off  mode=Lower Bit Location + Width  bit1=0  base1=MSB of Input  bit0=0  base0=LSB of Input  dbl_ovrd=off  block_type=slice
  nota{1..2,5..7} (5 alike) : xbsIndex_r4/Constant  const=0  gui_display_data_type=Fixed-point  arith_type=Unsigned  n_bits=7  bin_pt=0  preci_type=Single  exp_width=8  frac_width=24  explicit_period=on  period=1  equ=P=C  opselect=C  inp2=PCIN>>17  opr=+  inp1=P  carry=CIN  dbl_ovrd=off  block_type=constant
      settings: block_version=VER_STRING_GOES_HERE
  nota4 : xbsIndex_r4/Constant  const=44  gui_display_data_type=Fixed-point  arith_type=Unsigned  n_bits=7  bin_pt=0  preci_type=Single  exp_width=8  frac_width=24  explicit_period=on  period=1  equ=P=C  opselect=C  inp2=PCIN>>17  opr=+  inp1=P  carry=CIN  dbl_ovrd=off  block_type=constant
      settings: block_version=VER_STRING_GOES_HERE
  prg3 : xbsIndex_r4/Delay  rst=off  infoeditControl=Selection of Reset will increase slice count due to use of real FFs and instead of SRLs  en=off  latency=10  reg_retiming=on  dbl_ovrd=off  block_type=delay
      settings: block_version=8.2-EVAL
  vol{1..2,4..6} (5 alike) : xbsIndex_r4/Constant  const=0  gui_display_data_type=Fixed-point  arith_type=Unsigned  n_bits=8  bin_pt=0  preci_type=Single  exp_width=8  frac_width=24  explicit_period=on  period=1  equ=P=C  opselect=C  inp2=PCIN>>17  opr=+  inp1=P  carry=CIN  dbl_ovrd=off  block_type=constant
      settings: block_version=VER_STRING_GOES_HERE
  vol3 : xbsIndex_r4/Constant  const=100  gui_display_data_type=Fixed-point  arith_type=Unsigned  n_bits=8  bin_pt=0  preci_type=Single  exp_width=8  frac_width=24  explicit_period=on  period=1  equ=P=C  opselect=C  inp2=PCIN>>17  opr=+  inp1=P  carry=CIN  dbl_ovrd=off  block_type=constant
      settings: block_version=VER_STRING_GOES_HERE
  vol : Outport  VectorParamsAs1DForOutWhenUnconnected=off
  nota : Outport  Port=2  VectorParamsAs1DForOutWhenUnconnected=off
  en : Outport  Port=3  VectorParamsAs1DForOutWhenUnconnected=off
  wires:
  Register1/1 -> Counter/1
  Constant10/1 -> Register1/1
  Relational3/1 -> Register1/2
  Constant3/1 -> Relational3/2
  Counter1/1 -> Relational3/1
  Concat6/1 -> Mux1/5
  vol2/1 -> Concat6/1
  nota2/1 -> Concat6/2
  Concat1/1 -> Mux1/7
  vol6/1 -> Concat1/1
  nota1/1 -> Concat1/2
  Concat5/1 -> Mux1/6
  Relational2/1 -> Logical3/6
  Relational1/1 -> Logical3/5
  Constant2/1 -> Relational2/1
  Constant1/1 -> Relational1/1
  Counter/1 -> Relational2/2, Relational1/2, Relational11/2, Relational12/2, Relational9/2, Relational10/2, Relational13/2
  Constant4/1 -> Accumulator/1
  Logical3/1 -> Accumulator/2, Logical7/1
  Constant5/1 -> Relational9/1
  Constant6/1 -> Relational10/1
  Constant7/1 -> Relational12/1
  Constant8/1 -> Relational11/1
  Relational9/1 -> Logical3/1
  Relational10/1 -> Logical3/2
  Relational12/1 -> Logical3/3
  Relational11/1 -> Logical3/4
  Accumulator/1 -> Mux1/1
  vol3/1 -> Concat2/1
  nota4/1 -> Concat2/2
  vol4/1 -> Concat3/1
  nota5/1 -> Concat3/2
  vol1/1 -> Concat4/1
  nota6/1 -> Concat4/2
  vol5/1 -> Concat5/1
  nota7/1 -> Concat5/2
  Concat2/1 -> Mux1/2
  Concat3/1 -> Mux1/3
  Concat4/1 -> Mux1/4
  Mux1/1 -> Slice3/1, Slice2/1
  Constant9/1 -> Relational13/1
  Relational13/1 -> Logical7/2
  Logical7/1 -> prg3/1
  Slice2/1 -> vol/1
  Slice3/1 -> nota/1
  prg3/1 -> en/1

== system test_mashinka_mapp_4/ci_re_9 ==
  addr : Inport
  m_data : Inport  Port=2
  m_addr : Inport  Port=3
  m_en : Inport  Port=4
  Convert2 : xbsIndex_r4/Convert  gui_display_data_type=Floating-point  arith_type=Floating-point  n_bits=16  bin_pt=14  float_type=Single  exp_bits=8  fraction_bits=24  quantization=Truncate  overflow=Wrap  en=off  latency=6  pipeline=off  dbl_ovrd=off  block_type=convert
  Delay{1..5} (5 alike) : xbsIndex_r4/Delay  rst=off  infoeditControl=Selection of Reset will increase slice count due to use of real FFs and instead of SRLs  en=off  latency=1  reg_retiming=off  dbl_ovrd=off  block_type=delay
  Delay6 : xbsIndex_r4/Delay  rst=off  infoeditControl=Selection of Reset will increase slice count due to use of real FFs and instead of SRLs  en=off  latency=1  reg_retiming=on  dbl_ovrd=off  block_type=delay
      settings: xl_area=[16 32 0 0 0 0 0]  block_version=VER_STRING_GOES_HERE
  Delay7 : xbsIndex_r4/Delay  rst=off  infoeditControl=Selection of Reset will increase slice count due to use of real FFs and instead of SRLs  en=off  latency=1  reg_retiming=on  dbl_ovrd=off  block_type=delay
      settings: xl_area=[16 32 0 0 0 0 0]  block_version=VER_STRING_GOES_HERE
  Mux1 : xbsIndex_r4/Mux  inputs=2  en=off  latency=0  precision=Full  arith_type=Unsigned  n_bits=16  bin_pt=14  quantization=Truncate  overflow=Wrap  dbl_ovrd=off  block_type=mux
  RSlice1 : xbsIndex_r4/Slice  nbits=9  boolean_output=off  mode=Lower Bit Location + Width  bit1=0  base1=MSB of Input  bit0=0  base0=LSB of Input  dbl_ovrd=off  block_type=slice
      settings: block_version=VER_STRING_GOES_HERE
  Reinterpret2 : xbsIndex_r4/Reinterpret  force_arith_type=on  arith_type=Unsigned  force_bin_pt=on  bin_pt=0  block_type=reinterpret
  Reinterpret9 : xbsIndex_r4/Reinterpret  force_arith_type=on  arith_type=Floating-point  force_bin_pt=on  bin_pt=24  block_type=reinterpret
  Relational14 : xbsIndex_r4/Relational  mode=a=b  op_type=Bool  en=off  latency=0  dbl_ovrd=off  block_type=relational
  Single Port RAM2 : xbsIndex_r4/Single Port RAM  depth=512  initVector=[Res Res]  distributed_mem=Block RAM  write_mode=Read After Write  rst=off  init_reg=0  en=off  optimize_latency=off  latency=1  optimize=Area  dbl_ovrd=off  simulation_type=fast_sim  block_type=spram
  re_0 : xbsIndex_r4/Constant  const=CMD_ci_Re_9  gui_display_data_type=Fixed-point  arith_type=Unsigned  n_bits=8  bin_pt=0  preci_type=Single  exp_width=8  frac_width=24  explicit_period=on  period=1  equ=P=C  opselect=C  inp2=PCIN>>17  opr=+  inp1=P  carry=CIN  dbl_ovrd=off  block_type=constant
      settings: block_version=VER_STRING_GOES_HERE
  Out : Outport  VectorParamsAs1DForOutWhenUnconnected=off
  wires:
  Delay5/1 -> Single Port RAM2/3, Mux1/1
  Delay1/1 -> Single Port RAM2/2
  Delay4/1 -> Out/1
  Single Port RAM2/1 -> Delay2/1
  Convert2/1 -> Delay4/1
  Delay2/1 -> Reinterpret9/1
  Reinterpret9/1 -> Delay3/1
  Delay3/1 -> Convert2/1
  Mux1/1 -> Single Port RAM2/1
  re_0/1 -> Relational14/2
  Relational14/1 -> Delay5/1
  addr/1 -> Mux1/2
  m_en/1 -> Relational14/1
  m_data/1 -> Delay1/1
  RSlice1/1 -> Delay7/1
  Delay7/1 -> Reinterpret2/1
  Reinterpret2/1 -> Delay6/1
  m_addr/1 -> RSlice1/1
  Delay6/1 -> Mux1/3

== system test_mashinka_mapp_4/en1 ==
  In1 : Inport
  Delay : xbsIndex_r4/Delay  rst=off  infoeditControl=Selection of Reset will increase slice count due to use of real FFs and instead of SRLs  en=off  latency=1  reg_retiming=off  dbl_ovrd=off  block_type=delay
  Logical : xbsIndex_r4/Logical  logical_function=AND  inputs=2  en=off  latency=0  precision=Full  arith_type=Unsigned  n_bits=16  bin_pt=0  align_bp=on  dbl_ovrd=off  block_type=logical
  Logical1 : xbsIndex_r4/Logical  logical_function=XOR  inputs=2  en=off  latency=0  precision=Full  arith_type=Unsigned  n_bits=16  bin_pt=0  align_bp=on  dbl_ovrd=off  block_type=logical
  Out1 : Outport  VectorParamsAs1DForOutWhenUnconnected=off
  wires:
  In1/1 -> Logical/1, Delay/1, Logical1/2
  Logical/1 -> Out1/1
  Delay/1 -> Logical1/1
  Logical1/1 -> Logical/2

== system test_mashinka_mapp_4/en2 ==
  In1 : Inport
  Delay : xbsIndex_r4/Delay  rst=off  infoeditControl=Selection of Reset will increase slice count due to use of real FFs and instead of SRLs  en=off  latency=1  reg_retiming=off  dbl_ovrd=off  block_type=delay
  Logical : xbsIndex_r4/Logical  logical_function=AND  inputs=2  en=off  latency=0  precision=Full  arith_type=Unsigned  n_bits=16  bin_pt=0  align_bp=on  dbl_ovrd=off  block_type=logical
  Logical1 : xbsIndex_r4/Logical  logical_function=XOR  inputs=2  en=off  latency=0  precision=Full  arith_type=Unsigned  n_bits=16  bin_pt=0  align_bp=on  dbl_ovrd=off  block_type=logical
  Out1 : Outport  VectorParamsAs1DForOutWhenUnconnected=off
  wires:
  Logical1/1 -> Logical/2
  Delay/1 -> Logical1/1
  Logical/1 -> Out1/1
  In1/1 -> Logical1/2, Delay/1, Logical/1

== system test_mashinka_mapp_4/mashinka_0 ==
  Addr_param : Inport
  Dat_param : Inport  Port=2
  we_param : Inport  Port=3
  Addr : Inport  Port=4
  force : Inport  Port=5
  NN : Inport  Port=6
  Pedal : Inport  Port=7
  Reset : Inport  Port=8
  start : Inport  Port=9
  nn_fl : Inport  Port=10
  LASTX0 : Inport  Port=11
  LASTX1 : Inport  Port=12
  LASTX2 : Inport  Port=13
  LASTX3 : Inport  Port=14
  Constant1 : xbsIndex_r4/Constant  const=0  gui_display_data_type=Floating-point  arith_type=Floating-point  n_bits=16  bin_pt=14  preci_type=Single  exp_width=8  frac_width=24  explicit_period=on  period=1  equ=P=C  opselect=C  inp2=PCIN>>17  opr=+  inp1=P  carry=CIN  dbl_ovrd=off  block_type=constant
  Force_str0 : Subsystem  mask{num_str_12=num_str0, num_point_256=num_pts0, num_param=9, num_harm_32=num_harm_0}
      mask prompts: num_str_12 "num of strings"; num_point_256 "num of points"; num_param "num param"; num_harm_32 "num harms"
  RSlice4 : xbsIndex_r4/Slice  nbits=24  boolean_output=off  mode=Lower Bit Location + Width  bit1=0  base1=MSB of Input  bit0=0  base0=LSB of Input  dbl_ovrd=off  block_type=slice
      settings: block_version=VER_STRING_GOES_HERE
  Register{1,68..75} (9 alike) : xbsIndex_r4/Register  init=0  rst=off  en=off  dbl_ovrd=off  block_type=register
  Reinterpret2 : xbsIndex_r4/Reinterpret  force_arith_type=on  arith_type=Unsigned  force_bin_pt=on  bin_pt=0  block_type=reinterpret
  out_0 : Outport  VectorParamsAs1DForOutWhenUnconnected=off
  out_1 : Outport  Port=2  VectorParamsAs1DForOutWhenUnconnected=off
  out_2 : Outport  Port=3  VectorParamsAs1DForOutWhenUnconnected=off
  out_3 : Outport  Port=4  VectorParamsAs1DForOutWhenUnconnected=off
  wires:
  Force_str0/4(Force_nota3) -> out_3/1
  Force_str0/3(Force_nota2) -> out_2/1
  Force_str0/2(Force_nota1) -> out_1/1
  Force_str0/1(Force_nota0) -> out_0/1
  Register1/1 -> Force_str0/10(nn_fl)
  nn_fl/1 -> Register1/1
  start/1 -> Force_str0/9(start)
  RSlice4/1 -> Reinterpret2/1
  Register71/1 -> Force_str0/7(Pedal)
  Register68/1 -> Force_str0/1(Force_in)
  Register73/1 -> Force_str0/2(NN_in)
  Register70/1 -> Force_str0/8(Reset)
  Register74/1 -> Force_str0/5(Dat_param)
  Register69/1 -> Force_str0/3(Addr)
  Register75/1 -> Force_str0/4(Addr_param)
  Register72/1 -> Force_str0/6(we_param)
  NN/1 -> Register73/1
  Pedal/1 -> Register71/1
  we_param/1 -> Register72/1
  force/1 -> Register68/1
  Reset/1 -> Register70/1
  Addr/1 -> Register69/1
  Dat_param/1 -> RSlice4/1
  Addr_param/1 -> Register75/1
  Reinterpret2/1 -> Register74/1
  LASTX0/1 -> Force_str0/11(LASTX0)
  LASTX3/1 -> Force_str0/14(LASTX3)
  LASTX1/1 -> Force_str0/12(LASTX1)
  LASTX2/1 -> Force_str0/13(LASTX2)
